simulink model "DAB_Converter_D1"  (R2024a)
settings: Solver=VariableStepAuto  StartTime=0.0  StopTime=0.05  RelTol=1e-3
libraries: spsMosfetLib x8, spsCurrentMeasurementLib x3, spsDCVoltageSourceLib x2, spsVoltageMeasurementLib x2, spsLinearTransformerLib x1, spsMeanLib x1, spsRMSLib x1, spsSeriesRLCBranchLib x1, spspowerguiLib x1
settings Model: Creator=abhik  LastModifiedBy=abhik

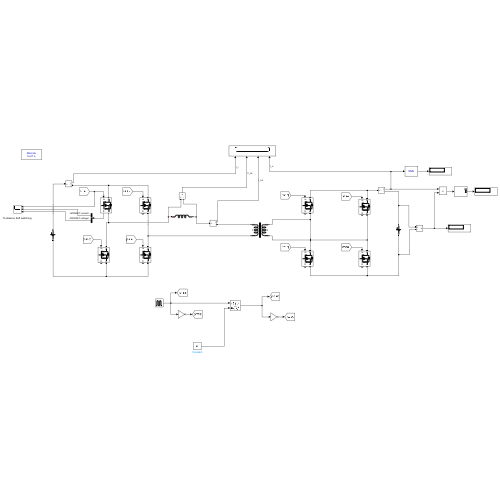
[thumbnail: Simulink's stored preview of the top-level diagram]
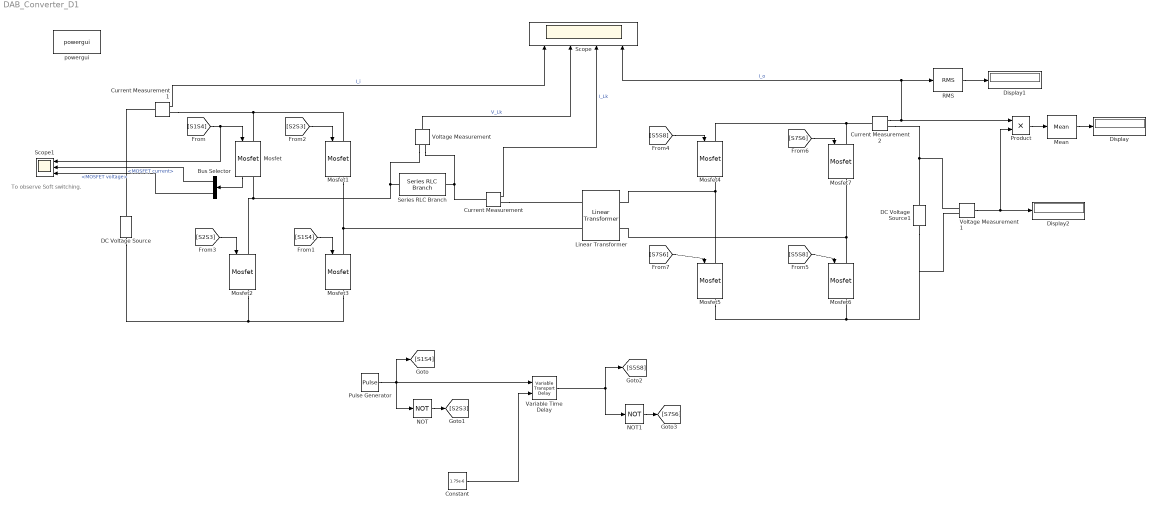
== system DAB_Converter_D1 ==
  note: To observe Soft switching.
  Bus Selector : BusSelector  OutputSignals=MOSFET current,MOSFET voltage
  Constant : Constant  Value=1.75e-6
  Current Measurement : spsCurrentMeasurementLib/Current Measurement  PhasorSimulation=off  OutputType=Complex  PSBequivalent=0
  Current Measurement1 : spsCurrentMeasurementLib/Current Measurement  PhasorSimulation=off  OutputType=Complex  PSBequivalent=0
  Current Measurement2 : spsCurrentMeasurementLib/Current Measurement  PhasorSimulation=off  OutputType=Complex  PSBequivalent=0
  DC Voltage Source : spsDCVoltageSourceLib/DC Voltage Source  Amplitude=48  Measurements=None
  DC Voltage Source1 : spsDCVoltageSourceLib/DC Voltage Source  Amplitude=400  Measurements=None
  Display : Display
  Display1 : Display
  Display2 : Display
  Linear Transformer : spsLinearTransformerLib/Linear Transformer  UNITS=SI  NominalPower=[ 1000 100e3]  winding1=[48 0 0]  winding2=[384 0 0]  ThreeWindings=off  winding3=[3.15e+05 0.7938 0.084225]  RmLm=[1.0804e+06 2866]  Measurements=None  DataType=on
  Mean : spsMeanLib/Mean  Freq=60  Vinit=0  Ts=0
  Mosfet{,1..7} (8 alike) : spsMosfetLib/Mosfet  Ron=0.1  Lon=0  Rd=0.01  Vfd=0  IC=0  Rs=1e5  Cs=inf  Measurements=on
  NOT : Logic  Operator=NOT  IconShape=distinctive  AllPortsSameDT=off  OutDataTypeStr=boolean
  NOT1 : Logic  Operator=NOT  IconShape=distinctive  AllPortsSameDT=off  OutDataTypeStr=boolean
  Product : Product
  Pulse Generator : DiscretePulseGenerator  PulseType=Time based  Period=1e-5  PulseWidth=50
  RMS : spsRMSLib/RMS  TrueRMS=on  Freq=60  RMSInit=120  Ts=0
  Scope : Scope  NumInputPorts=4
  Scope1 : Scope  NumInputPorts=3
  Series RLC Branch : spsSeriesRLCBranchLib/Series RLC Branch  LConnTagsString=__new0  RConnTagsString=__new0  BranchType=L  Resistance=1  Inductance=2.62e-6  SetiL0=off  InitialCurrent=0  Capacitance=1e-6  Setx0=off  InitialVoltage=0  Measurements=None
  Variable Time Delay : VariableTransportDelay  MaximumDelay=10
  Voltage Measurement : spsVoltageMeasurementLib/Voltage Measurement  PhasorSimulation=off  OutputType=Complex  PSBequivalent=0
  Voltage Measurement1 : spsVoltageMeasurementLib/Voltage Measurement  PhasorSimulation=off  OutputType=Complex  PSBequivalent=0
  powergui : spspowerguiLib/powergui  Priority=1  SimulationMode=Discrete  SampleTime=1e-7  frequency=60  Iterations=50  frequencyindice=0  Pbase=100e6  ErrMax=1e-4  UnitsV=kV  UnitsW=MW  buscounter=0  FunctionMessages=off  echomessages=off  EnableUseOfTLC=off  CurrentSourceSwitches=off  DisableSnubberDevices=off  DisableRonSwitches=off  DisableVfSwitches=off  DisplayEquations=off  AutomaticDiscreteSolvers=off  SolverType=Tustin/Backward Euler (TBE)  Interpol=off  ExternalGateDelay=off  methode=off  Ts=100  x0status=blocks  SPID=on  SwTol=0  HookPort=off  NonlinearTolerance=1e-4  nMaxIteration=100  ContinueOnMaxIteration=off  RestoreLinks=warning  ResistiveCurrentMeasurement=off  Frange=[0:2:500]  Ylog=off  Xlog=on  ShowGrid=off  save=off  variable=ZData  structure=0  ZoomFFT=off  StartTime=0.0  cycles=1  DisplayStyle=1  fundamental=60  FreqAxis=off  MaxFrequency=1000  frequencyindicesteady=1  RmsSteady=1  display=off
  wires:
  Pulse Generator/1 -> [S1S4], Variable Time Delay/1, NOT/1
  [S1S4] -> Scope1/1, Mosfet/1
  [S1S4] -> Mosfet3/1
  NOT/1 -> [S2S3]
  [S2S3] -> Mosfet1/1
  [S2S3] -> Mosfet2/1
  [S5S8] -> Mosfet4/1
  [S7S6] -> Mosfet7/1
  [S5S8] -> Mosfet6/1
  Variable Time Delay/1 -> [S5S8], NOT1/1
  NOT1/1 -> [S7S6]
  Voltage Measurement/1 -> Scope/2  "V_Lk"
  Current Measurement/1 -> Scope/3  "I_Lk"
  [S7S6] -> Mosfet5/1
  Current Measurement1/1 -> Scope/1  "I_i"
  Current Measurement2/1 -> RMS/1, Scope/4, Product/1  "I_o"
  Mosfet/1 -> Bus Selector/1
  Bus Selector/1 -> Scope1/2  "<MOSFET current>"
  Bus Selector/2 -> Scope1/3  "<MOSFET voltage>"
  Voltage Measurement1/1 -> Display2/1, Product/2
  Product/1 -> Mean/1
  Mean/1 -> Display/1
  RMS/1 -> Display1/1
  Constant/1 -> Variable Time Delay/2
  connections:
  DC Voltage Source/LConn1 -- Mosfet3/RConn1 -- Mosfet2/RConn1
  Series RLC Branch/LConn1 -- Mosfet2/LConn1 -- Mosfet/RConn1 -- Voltage Measurement/LConn1
  Mosfet1/RConn1 -- Linear Transformer/LConn2 -- Mosfet3/LConn1
  Current Measurement/RConn1 -- Linear Transformer/LConn1
  Mosfet4/LConn1 -- Mosfet7/LConn1 -- Current Measurement2/LConn1
  Mosfet5/LConn1 -- Linear Transformer/RConn1 -- Mosfet4/RConn1
  Mosfet6/LConn1 -- Mosfet7/RConn1 -- Linear Transformer/RConn2
  Mosfet5/RConn1 -- Voltage Measurement1/LConn2 -- DC Voltage Source1/LConn1 -- Mosfet6/RConn1
  Voltage Measurement/LConn2 -- Current Measurement/LConn1 -- Series RLC Branch/RConn1
  DC Voltage Source/RConn1 -- Current Measurement1/LConn1
  Mosfet1/LConn1 -- Current Measurement1/RConn1 -- Mosfet/LConn1
  Current Measurement2/RConn1 -- Voltage Measurement1/LConn1 -- DC Voltage Source1/RConn1
